simulink model "symbolic_test"  (Simulink 8.1)
settings: Solver=ode45  StartTime=0.0  StopTime=10.0  RelTol=1e-3
values from neighbouring files (symbols this model uses):
  a = p.Results    [TIPS_TRICKS.m]
  b = @(x,y) arrayfun(@(y)get,x,y)    [TIPS_TRICKS.m]    (also in UMTSb.m = 3)
  c = lambda/T    [EMW_d.m]
settings Model: Creator=mainster  LastModifiedBy=mainster
settings DataIOCC: SignalLoggingSaveFormat=Dataset
settings OptimizationCC: ExpressionDepthLimit=128
settings DebuggingCC: FcnCallInpInsideContextMsg=EnableAllAsError
settings GRTTargetCC: CombineOutputUpdateFcns=on  GRTInterface=off

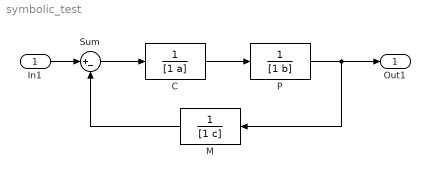
== system symbolic_test ==
  In1 : Inport
  C : TransferFcn  Denominator=[1 a]
  M : TransferFcn  Denominator=[1 c]
  P : TransferFcn  Denominator=[1 b]
  Sum : Sum  Inputs=|+-
  Out1 : Outport
  wires:
  C/1 -> P/1
  P/1 -> M/1, Out1/1
  In1/1 -> Sum/1
  Sum/1 -> C/1
  M/1 -> Sum/2
